simulink model "model2"  (R2019b)
settings: Solver=VariableStepAuto  StartTime=0.0  StopTime=1  RelTol=1e-3
libraries: simulink x2
settings Model: Creator=surtweig  LastModifiedBy=surtweig

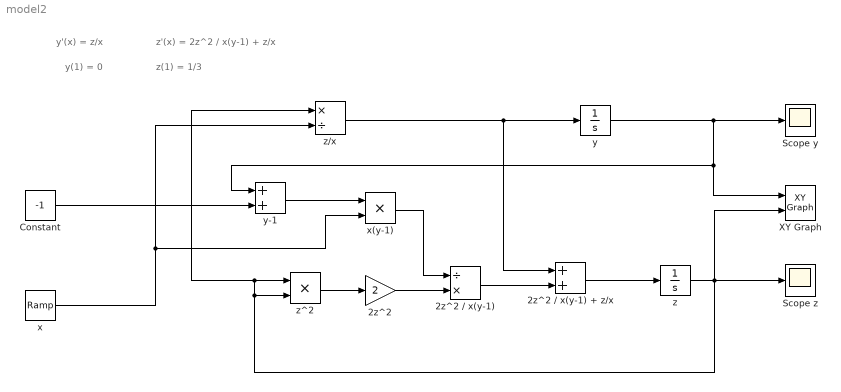
== system model2 ==
  note: z(1) = 1/3
  note: y(1) = 0
  note: z'(x) = 2z^2 / x(y-1) + z/x
  note: y'(x) = z/x
  2z^2 : Gain  Gain=2
  2z^2 / x(y-1) : Product  Inputs=/*
  2z^2 / x(y-1) + z/x : Sum
  Constant : Constant  Value=-1
  Scope y : Scope
  Scope z : Scope
  XY Graph : simulink/Sinks/XY Graph  xmin=-1  xmax=1  ymin=-1  ymax=1  st=-1
  x : simulink/Sources/Ramp  slope=1  start=0  InitialOutput=1
  x(y-1) : Product
  y : Integrator
  y-1 : Sum
  z : Integrator  InitialCondition=1/3
  z/x : Product  Inputs=*/
  z^2 : Product
  wires:
  x/1 -> x(y-1)/2, z/x/2
  z/x/1 -> 2z^2 / x(y-1) + z/x/1, y/1
  y/1 -> XY Graph/1, y-1/1, Scope y/1
  z^2/1 -> 2z^2/1
  2z^2 / x(y-1)/1 -> 2z^2 / x(y-1) + z/x/2
  2z^2 / x(y-1) + z/x/1 -> z/1
  2z^2/1 -> 2z^2 / x(y-1)/2
  x(y-1)/1 -> 2z^2 / x(y-1)/1
  y-1/1 -> x(y-1)/1
  Constant/1 -> y-1/2
  z/1 -> XY Graph/2, Scope z/1, z/x/1, z^2/1, z^2/2
